simulink subsystem "air_removal_control"  (R2022b)
settings: Solver=VariableStepAuto  StartTime=0.0  StopTime=1000  RelTol=1e-3
model mask{tank_max=500, pump_switch_time=300, valve_switch_time=300, tank_min=250, switch_tolerance_mm=50}
  mask prompts: tank_max "Tank maximum level [mm]"; pump_switch_time "Time between switch of aux pump [s]"; valve_switch_time "Time before consumer valve opens [s]"; tank_min "Tank_minimum_level [mm]"; switch_tolerance_mm "Forward or return max min tolerance [mm]"
settings Model: DefaultTestHarness=air_removal_control_Harness1  Creator=pppc  LastModifiedBy=pppc

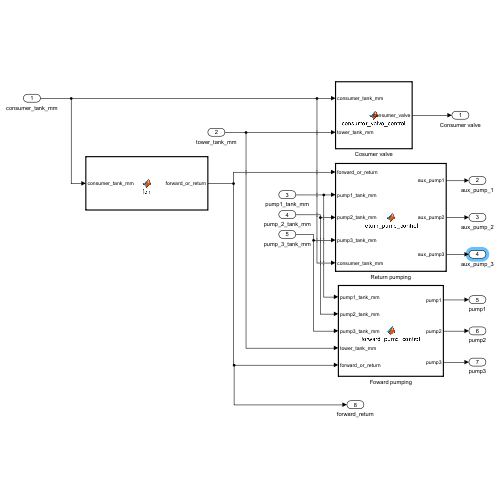
[thumbnail: Simulink's stored preview of the top-level diagram]
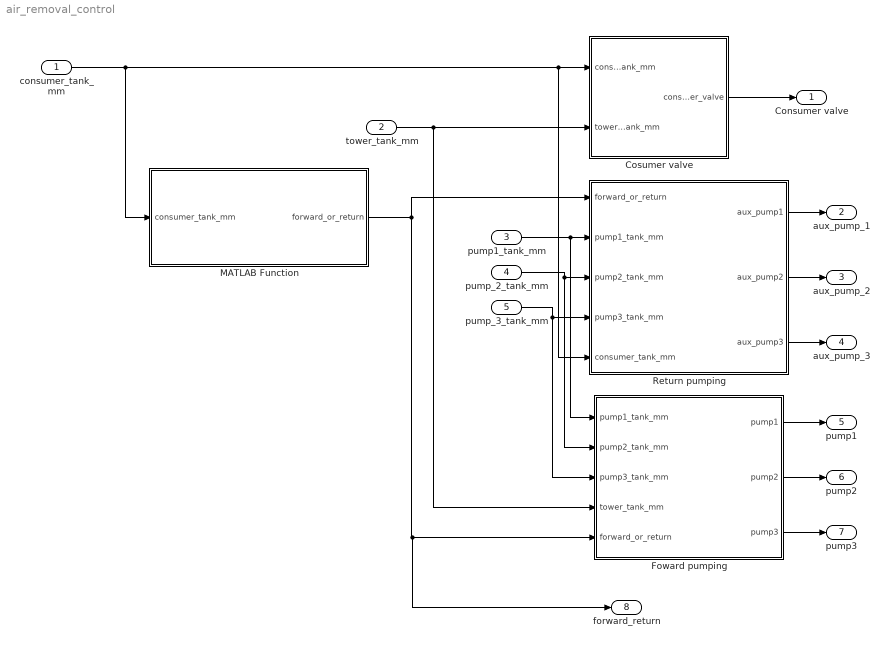
== system air_removal_control ==
  consumer_tank_mm : Inport
  tower_tank_mm : Inport  Port=2
  pump1_tank_mm : Inport  Port=3
  pump_2_tank_mm : Inport  Port=4
  pump_3_tank_mm : Inport  Port=5
  Cosumer valve : MATLAB Function  TreatAsAtomicUnit=on  SystemSampleTime=1
  Foward pumping : MATLAB Function  TreatAsAtomicUnit=on  SystemSampleTime=1
  MATLAB Function : MATLAB Function  TreatAsAtomicUnit=on
  Return pumping : MATLAB Function  TreatAsAtomicUnit=on  SystemSampleTime=1
  Consumer valve : Outport
  aux_pump_1 : Outport  Port=2
  aux_pump_2 : Outport  Port=3
  aux_pump_3 : Outport  Port=4
  pump1 : Outport  Port=5
  pump2 : Outport  Port=6
  pump3 : Outport  Port=7
  forward_return : Outport  Port=8
  wires:
  Return pumping/1(aux_pump1) -> aux_pump_1/1
  Return pumping/2(aux_pump2) -> aux_pump_2/1
  Foward pumping/3(pump3) -> pump3/1
  pump_2_tank_mm/1 -> Foward pumping/2(pump2_tank_mm), Return pumping/3(pump2_tank_mm)
  consumer_tank_mm/1 -> MATLAB Function/1(consumer_tank_mm), Return pumping/5(consumer_tank_mm), Cosumer valve/1(consumer_tank_mm)
  tower_tank_mm/1 -> Cosumer valve/2(tower_tank_mm), Foward pumping/4(tower_tank_mm)
  pump_3_tank_mm/1 -> Foward pumping/3(pump3_tank_mm), Return pumping/4(pump3_tank_mm)
  Cosumer valve/1(consumer_valve) -> Consumer valve/1
  Foward pumping/1(pump1) -> pump1/1
  Return pumping/3(aux_pump3) -> aux_pump_3/1
  pump1_tank_mm/1 -> Return pumping/2(pump1_tank_mm), Foward pumping/1(pump1_tank_mm)
  Foward pumping/2(pump2) -> pump2/1
  MATLAB Function/1(forward_or_return) -> Return pumping/1(forward_or_return), forward_return/1, Foward pumping/5(forward_or_return)

== matlab function air_removal_control/MATLAB Function ==
  data: consumer_tank_mm input; forward_or_return output; tank_min parameter; tank_max parameter; switch_tolerance_mm parameter
function forward_or_return = fcn(consumer_tank_mm,tank_min, tank_max, switch_tolerance_mm)
persistent forward_return_local
if(isempty(forward_return_local)); forward_return_local = 1; end

if(consumer_tank_mm<tank_min + switch_tolerance_mm)
    forward_return_local = 1;
end

if(consumer_tank_mm>tank_max - switch_tolerance_mm)
    forward_return_local = 0;
end 

forward_or_return = forward_return_local;

== matlab function air_removal_control/Cosumer valve ==
  data: consumer_tank_mm input; consumer_valve output; tower_tank_mm input; valve_switch_time parameter; tank_min parameter; tank_max parameter
function consumer_valve = consumer_valve_control(consumer_tank_mm, tower_tank_mm,valve_switch_time, tank_min, tank_max)
%Function to be called once every second
persistent close_time
if(isempty(close_time)); close_time = 0; end


consumer_valve = 0;
if(consumer_tank_mm > tank_max || tower_tank_mm < tank_min)
    consumer_valve = 0;
    close_time = 0;
    return
end

%Ensuer valve stay close for 3 minutes after the opening criteria is
%fulfilled
close_time = close_time + 1;
if(close_time > valve_switch_time)
    consumer_valve = 100;
    return
end

end

== matlab function air_removal_control/Foward pumping ==
  data: pump1_tank_mm input; pump2_tank_mm input; pump3_tank_mm input; tower_tank_mm input; forward_or_return input; pump1 output; pump2 output; pump3 output; tank_min parameter; tank_max parameter
function [pump1, pump2, pump3]= forward_pump_control(pump1_tank_mm, pump2_tank_mm, pump3_tank_mm, tower_tank_mm, forward_or_return, tank_min, tank_max)


pump1 = 100;
pump2 = 100;
pump3 = 100;

if(forward_or_return==false || tower_tank_mm > tank_max)
    pump1 = 0;
    pump2 = 0;
    pump3 = 0;
    return
end

%Turn off pumps if their tank is empty
if(pump1_tank_mm < tank_min)
    pump1=0;
end

if(pump2_tank_mm < tank_min)
    pump2=0;
end

if(pump3_tank_mm < tank_min)
    pump3=0;
end


end

== matlab function air_removal_control/Return pumping ==
  data: forward_or_return input; pump1_tank_mm input; pump2_tank_mm input; pump3_tank_mm input; consumer_tank_mm input; aux_pump1 output; aux_pump2 output; aux_pump3 output; tank_min parameter; tank_max parameter; pump_switch_time parameter
function [aux_pump1, aux_pump2, aux_pump3]= return_pump_control(forward_or_return, pump1_tank_mm, pump2_tank_mm, pump3_tank_mm, consumer_tank_mm, tank_min, tank_max, pump_switch_time)
% Fnction to be called once every second
persistent pump_run_time
if(isempty(pump_run_time)); pump_run_time=0; end

persistent pump_number
if(isempty(pump_number)); pump_number=1; end

aux_pump1 = 0;
aux_pump2 = 0;
aux_pump3 = 0;

% Check 
if(consumer_tank_mm < tank_min || forward_or_return == 1)
     return
end


switch pump_number
    case 1
        pump_run_time = pump_run_time  +1;
        if(pump_run_time > pump_switch_time || pump1_tank_mm > tank_max)
            pump_number = 2;
            pump_run_time = 0;
        else 
            aux_pump1 = 100;
        end
        
    case 2
        pump_run_time = pump_run_time  +1;
        if(pump_run_time > pump_switch_time || pump2_tank_mm > tank_max)
            pump_number = 3;
            pump_run_time = 0;
        else 
            aux_pump2 = 100;
        end

  case 3
        pump_run_time = pump_run_time  +1;
        if(pump_run_time > pump_switch_time || pump3_tank_mm > tank_max)
            pump_number = 1;
            pump_run_time = 0;
        else 
            aux_pump3 = 100;
        end
end
